simulink library "lib_tbm_presToTbFlag_whl"  (R2020a)
settings: Solver=VariableStepAuto  StartTime=0.0  StopTime=10.0  RelTol=1e-3
settings Model: Creator=Administrator  LastModifiedBy=Administrator

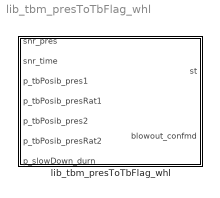
== system lib_tbm_presToTbFlag_whl ==
  lib_tbm_presToTbFlag_whl : Subsystem

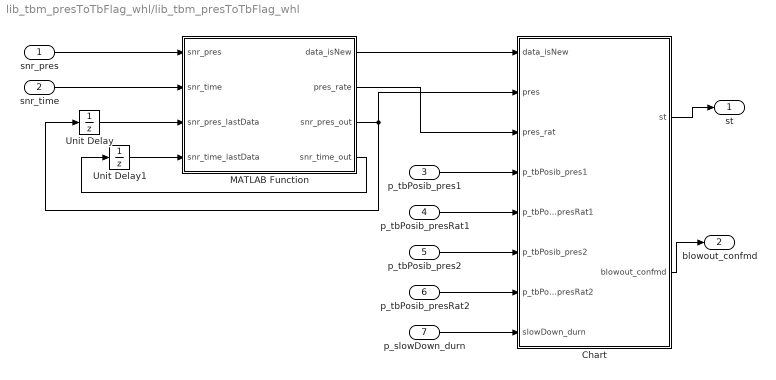
== system lib_tbm_presToTbFlag_whl/lib_tbm_presToTbFlag_whl ==
  snr_pres : Inport  OutDataTypeStr=single
  snr_time : Inport  Port=2  OutDataTypeStr=single
  p_tbPosib_pres1 : Inport  Port=3  OutDataTypeStr=single
  p_tbPosib_presRat1 : Inport  Port=4  OutDataTypeStr=single
  p_tbPosib_pres2 : Inport  Port=5  OutDataTypeStr=single
  p_tbPosib_presRat2 : Inport  Port=6  OutDataTypeStr=single
  p_slowDown_durn : Inport  Port=7
  Chart : Stateflow chart  TreatAsAtomicUnit=on
  MATLAB Function : MATLAB Function  TreatAsAtomicUnit=on
  Unit Delay : UnitDelay  SampleTime=-1  HasFrameUpgradeWarning=on
  Unit Delay1 : UnitDelay  SampleTime=-1  HasFrameUpgradeWarning=on
  st : Outport  OutDataTypeStr=uint8
  blowout_confmd : Outport  Port=2  OutDataTypeStr=boolean
  wires:
  snr_time/1 -> MATLAB Function/2(snr_time)
  MATLAB Function/3(snr_pres_out) -> Chart/2(pres), Unit Delay/1
  Unit Delay1/1 -> MATLAB Function/4(snr_time_lastData)
  MATLAB Function/2(pres_rate) -> Chart/3(pres_rat)
  Unit Delay/1 -> MATLAB Function/3(snr_pres_lastData)
  MATLAB Function/1(data_isNew) -> Chart/1(data_isNew)
  snr_pres/1 -> MATLAB Function/1(snr_pres)
  MATLAB Function/4(snr_time_out) -> Unit Delay1/1
  p_tbPosib_pres1/1 -> Chart/4(p_tbPosib_pres1)
  p_tbPosib_presRat1/1 -> Chart/5(p_tbPosib_presRat1)
  Chart/1(st) -> st/1
  Chart/2(blowout_confmd) -> blowout_confmd/1
  p_tbPosib_pres2/1 -> Chart/6(p_tbPosib_pres2)
  p_tbPosib_presRat2/1 -> Chart/7(p_tbPosib_presRat2)
  p_slowDown_durn/1 -> Chart/8(slowDown_durn)

== stateflow chart lib_tbm_presToTbFlag_whl/Chart ==
  state blowout_no
    en:
    st = 0;
    blowout_confmd = false;
  state blowout_possible
    en:
    st = 1;
    blowout_confmd = false;
  state blowout_comfirmed
    en:
    st = 2;
  state done
    en:
    st = 3;
    blowout_confmd = true;
  (default) -> blowout_no
  blowout_possible -> blowout_no [order 3] : after(0.1, sec)
  blowout_possible -> blowout_no [order 1] : [    ( pres > ( 1.2* p_tbPosib_pres1) ) ...
      |   || ( pres_rat >  0.5 * p_tbPosib_presRat2 ) ]
      | % p_rate is negative
  blowout_no -> (junction 10) : [data_isNew]
  (junction 10) -> blowout_possible [order 2] : [    ( pres < p_tbPosib_pres2) ...
      | && ( pres_rat < p_tbPosib_presRat2) ]
  (junction 10) -> blowout_possible [order 1] : [    ( pres < p_tbPosib_pres1) ...
      | && ( pres_rat < p_tbPosib_presRat1) ]
  blowout_possible -> (junction 18) [order 2] : [data_isNew]
  (junction 18) -> blowout_comfirmed [order 2] : [    ( pres < p_tbPosib_pres2) ...
      | && ( pres_rat < p_tbPosib_presRat2) ]
  (junction 18) -> blowout_comfirmed [order 1] : [    ( pres < p_tbPosib_pres1) ...
      | && ( pres_rat < p_tbPosib_presRat1) ]
  blowout_comfirmed -> done : after(slowDown_durn, sec)
  data: st output uint8; blowout_confmd output boolean; data_isNew input boolean; pres input single; pres_rat input; p_tbPosib_pres1 input single; p_tbPosib_presRat1 input single; p_tbPosib_pres2 input single; p_tbPosib_presRat2 input single; slowDown_durn input single

== matlab function lib_tbm_presToTbFlag_whl/MATLAB Function ==
  data: snr_pres input single; snr_time input single; data_isNew output boolean; snr_pres_lastData input single; snr_time_lastData input single; pres_rate output single; snr_pres_out output single; snr_time_out output single
function [data_isNew, pres_rate, snr_pres_out, snr_time_out] = fcn(snr_pres, snr_time, snr_pres_lastData, snr_time_lastData)

data_isNew = false; 
snr_pres_out = snr_pres_lastData;
snr_time_out = snr_time_lastData;
pres_rate = single(0);


if ( snr_time - snr_time_lastData )> 0.001     % sec
    data_isNew = true;   
    pres_rate = (snr_pres - snr_pres_lastData) / (snr_time - snr_time_lastData);
    snr_pres_out = snr_pres;
    snr_time_out = snr_time;
end
